simulink model "simulink_ex1"  (R2020a)
settings: Solver=FixedStepAuto  StartTime=0.0  StopTime=200  FixedStep=1e-3  RelTol=1e-3
settings Model: Creator=debora  LastModifiedBy=debora

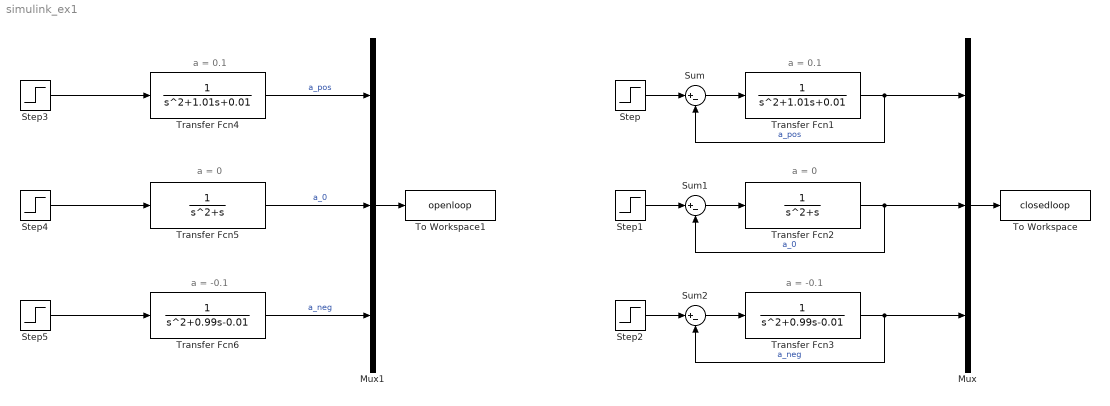
== system simulink_ex1 ==
  note: a = 0.1
  note: a = 0
  note: a = -0.1
  note: a = -0.1
  note: a = 0
  note: a = 0.1
  Mux : Mux  Inputs=3
  Mux1 : Mux  Inputs=3
  Step{,1..5} (6 alike) : Step  Time=0  SampleTime=0
  Sum : Sum  Inputs=|+-
  Sum1 : Sum  Inputs=|+-
  Sum2 : Sum  Inputs=|+-
  To Workspace : ToWorkspace  VariableName=closedloop  SaveFormat=Timeseries  SampleTime=-1
  To Workspace1 : ToWorkspace  VariableName=openloop  SaveFormat=Timeseries  SampleTime=-1
  Transfer Fcn1 : TransferFcn  Denominator=[1 1.01 0.01]
  Transfer Fcn2 : TransferFcn  Denominator=[1 1 0]
  Transfer Fcn3 : TransferFcn  Denominator=[1 0.99 -0.01]
  Transfer Fcn4 : TransferFcn  Denominator=[1 1.01 0.01]
  Transfer Fcn5 : TransferFcn  Denominator=[1 1 0]
  Transfer Fcn6 : TransferFcn  Denominator=[1 0.99 -0.01]
  wires:
  Sum/1 -> Transfer Fcn1/1
  Step/1 -> Sum/1
  Transfer Fcn1/1 -> Sum/2, Mux/1  "a_pos"
  Step1/1 -> Sum1/1
  Transfer Fcn2/1 -> Sum1/2, Mux/2  "a_0"
  Sum1/1 -> Transfer Fcn2/1
  Step2/1 -> Sum2/1
  Transfer Fcn3/1 -> Sum2/2, Mux/3  "a_neg"
  Sum2/1 -> Transfer Fcn3/1
  Mux/1 -> To Workspace/1
  Transfer Fcn6/1 -> Mux1/3  "a_neg"
  Step5/1 -> Transfer Fcn6/1
  Step3/1 -> Transfer Fcn4/1
  Step4/1 -> Transfer Fcn5/1
  Transfer Fcn4/1 -> Mux1/1  "a_pos"
  Transfer Fcn5/1 -> Mux1/2  "a_0"
  Mux1/1 -> To Workspace1/1
